simulink model "ExampleDPWM"  (R2023b)
settings: Solver=VariableStepAuto  StartTime=0.0  StopTime=0.1  FixedStep=50e-6  RelTol=1e-3
libraries: spsMosfetLib x6, spsSeriesRLCBranchLib x3, spsDCVoltageSourceLib x1, spsGroundLib x1, simulink_extras x1, spsThreePhaseVIMeasurementLib x1, spsTriangleGeneratorLib x1, spsVoltageMeasurementLib x1, sps_lib x1
settings Model: Creator=user  LastModifiedBy=user
settings DataIOCC: ReturnWorkspaceOutputs=off

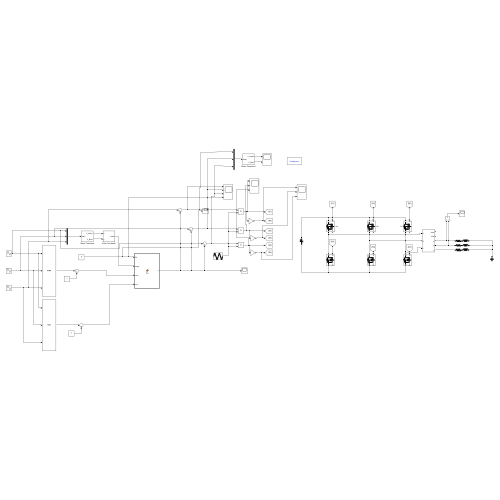
[thumbnail: Simulink's stored preview of the top-level diagram]
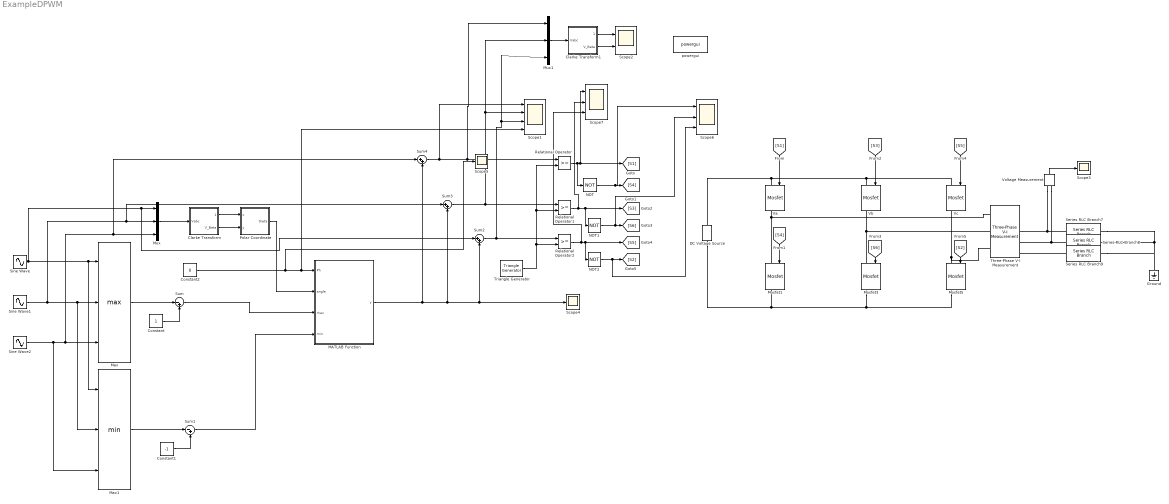
== system ExampleDPWM ==
  Clarke Transform : Subsystem
  Clarke Transform1 : Subsystem
  Constant : Constant
  Constant1 : Constant  Value=-1
  Constant2 : Constant  Value=0
  DC Voltage Source : spsDCVoltageSourceLib/DC Voltage Source  Amplitude=100  Measurements=None
  Ground : spsGroundLib/Ground  LConnTagsString=a
  MATLAB Function : MATLAB Function  TreatAsAtomicUnit=on
  Max : MinMax  Function=max  Inputs=3
  Max1 : MinMax  Inputs=3
  Mosfet1 : spsMosfetLib/Mosfet  Ron=0.1  Lon=0  Rd=0.01  Vfd=0  IC=0  Rs=1e5  Cs=inf  Measurements=on
  Mosfet3 : spsMosfetLib/Mosfet  Ron=0.1  Lon=0  Rd=0.01  Vfd=0  IC=0  Rs=1e5  Cs=inf  Measurements=on
  Mosfet5 : spsMosfetLib/Mosfet  Ron=0.1  Lon=0  Rd=0.01  Vfd=0  IC=0  Rs=1e5  Cs=inf  Measurements=on
  Mux : Mux  Inputs=3
  Mux1 : Mux  Inputs=3
  NOT : Logic  Operator=NOT  IconShape=distinctive  AllPortsSameDT=off  OutDataTypeStr=boolean
  NOT1 : Logic  Operator=NOT  IconShape=distinctive  AllPortsSameDT=off  OutDataTypeStr=boolean
  NOT2 : Logic  Operator=NOT  IconShape=distinctive  AllPortsSameDT=off  OutDataTypeStr=boolean
  Polar Coordinate : Subsystem
  Relational Operator : RelationalOperator  OutDataTypeStr=boolean  RndMeth=Simplest  InputSameDT=off
  Relational Operator1 : RelationalOperator  OutDataTypeStr=boolean  RndMeth=Simplest  InputSameDT=off
  Relational Operator2 : RelationalOperator  OutDataTypeStr=boolean  RndMeth=Simplest  InputSameDT=off
  Scope1 : Scope  NumInputPorts=4
  Scope2 : Scope  NumInputPorts=2
  Scope3 : Scope
  Scope4 : Scope
  Scope5 : Scope
  Scope6 : Scope  NumInputPorts=3
  Scope7 : Scope  NumInputPorts=3
  Series RLC Branch7 : spsSeriesRLCBranchLib/Series RLC Branch  LConnTagsString=__new0  RConnTagsString=__new0  BranchType=RL  Resistance=15  Inductance=10e-2  SetiL0=off  InitialCurrent=0  Capacitance=50e-6  Setx0=off  InitialVoltage=0  Measurements=None
  Series RLC Branch8 : spsSeriesRLCBranchLib/Series RLC Branch  LConnTagsString=__new0  RConnTagsString=__new0  BranchType=RL  Resistance=15  Inductance=10e-2  SetiL0=off  InitialCurrent=0  Capacitance=50e-6  Setx0=off  InitialVoltage=0  Measurements=None
  Series RLC Branch9 : spsSeriesRLCBranchLib/Series RLC Branch  LConnTagsString=__new0  RConnTagsString=__new0  BranchType=RL  Resistance=15  Inductance=10e-2  SetiL0=off  InitialCurrent=0  Capacitance=50e-6  Setx0=off  InitialVoltage=0  Measurements=None
  Sine Wave : Sin  Frequency=2*pi*50  SampleTime=0
  Sine Wave1 : Sin  Frequency=2*pi*50  Phase=(2*pi/3)  SampleTime=0
  Sine Wave2 : Sin  Frequency=2*pi*50  Phase=-2*pi/3  SampleTime=0
  Sum : Sum  Inputs=|-+
  Sum1 : Sum  Inputs=|-+
  Sum2 : Sum  Inputs=|++
  Sum3 : Sum  Inputs=|++
  Sum4 : Sum  Inputs=|++
  Three-Phase V-I Measurement : spsThreePhaseVIMeasurementLib/Three-Phase V-I Measurement  VoltageMeasurement=phase-to-phase  SetLabelV=off  LabelV=Vabc  Vpu=off  VpuLL=off  CurrentMeasurement=yes  SetLabelI=off  LabelI=Iabc  Ipu=off  Pbase=100e6  Vbase=500e3  OutputType=Complex  PhasorSimulation=off  PSBequivalent=0
  Triangle Generator : spsTriangleGeneratorLib/Triangle Generator  Freq=4000  Phase=90  Ts=0
  Va : spsMosfetLib/Mosfet  Ron=0.1  Lon=0  Rd=0.01  Vfd=0  IC=0  Rs=1e5  Cs=inf  Measurements=on
  Vb : spsMosfetLib/Mosfet  Ron=0.1  Lon=0  Rd=0.01  Vfd=0  IC=0  Rs=1e5  Cs=inf  Measurements=on
  Vc : spsMosfetLib/Mosfet  Ron=0.1  Lon=0  Rd=0.01  Vfd=0  IC=0  Rs=1e5  Cs=inf  Measurements=on
  Voltage Measurement : spsVoltageMeasurementLib/Voltage Measurement  PhasorSimulation=off  OutputType=Complex  PSBequivalent=0
  powergui : sps_lib/powergui  Priority=1  SimulationMode=Continuous  SampleTime=50e-6  frequency=60  Iterations=50  frequencyindice=0  Pbase=100e6  ErrMax=1e-4  UnitsV=kV  UnitsW=MW  buscounter=0  FunctionMessages=off  echomessages=off  EnableUseOfTLC=off  CurrentSourceSwitches=off  DisableSnubberDevices=off  DisableRonSwitches=off  DisableVfSwitches=off  DisplayEquations=off  AutomaticDiscreteSolvers=off  SolverType=Tustin/Backward Euler (TBE)  Interpol=off  ExternalGateDelay=off  methode=off  Ts=100  x0status=blocks  SPID=on  SwTol=0  HookPort=off  NonlinearTolerance=1e-4  nMaxIteration=100  ContinueOnMaxIteration=off  RestoreLinks=warning  ResistiveCurrentMeasurement=off  Frange=[0:2:500]  Ylog=off  Xlog=on  ShowGrid=off  save=off  variable=ZData  structure=0  ZoomFFT=off  StartTime=0.0  cycles=1  DisplayStyle=1  fundamental=60  FreqAxis=off  MaxFrequency=1000  frequencyindicesteady=1  RmsSteady=1  display=off
  wires:
  Sine Wave1/1 -> Sum3/1, Mux/2, Max1/2, Max/2
  Sine Wave2/1 -> Max1/3, Sum4/1, Mux/3, Max/3
  Max/1 -> Sum/1
  Constant/1 -> Sum/2
  Constant1/1 -> Sum1/2
  Max1/1 -> Sum1/1
  Clarke Transform/1(V_Alpha) -> Polar Coordinate/1(x)
  Clarke Transform/2(V_Beta) -> Polar Coordinate/2(y)
  Sine Wave/1 -> Sum2/1, Mux/1, Max1/1, Max/1
  Mux/1 -> Clarke Transform/1(Vabc)
  Polar Coordinate/1(theta) -> MATLAB Function/2(angle)
  Sum/1 -> MATLAB Function/3(max)
  Sum1/1 -> MATLAB Function/4(min)
  Sum3/1 -> Mux1/2, Scope1/2, Relational Operator1/1
  [S4] -> Mosfet1/1
  [S1] -> Va/1
  [S3] -> Vb/1
  [S2] -> Mosfet5/1
  [S5] -> Vc/1
  [S6] -> Mosfet3/1
  Relational Operator1/1 -> Scope7/2, [S3], NOT1/1
  Relational Operator2/1 -> Scope7/3, [S5], NOT2/1
  Triangle Generator/1 -> Relational Operator2/2, Relational Operator/2, Relational Operator1/2
  Relational Operator/1 -> Scope7/1, [S1], NOT/1
  Sum2/1 -> Mux1/3, Scope1/3, Relational Operator2/1
  NOT/1 -> Scope6/1, [S4]
  NOT1/1 -> Scope6/2, [S6]
  NOT2/1 -> Scope6/3, [S2]
  MATLAB Function/1(y) -> Sum4/2, Sum3/2, Sum2/2, Scope4/1
  Mux1/1 -> Clarke Transform1/1(Vabc)
  Clarke Transform1/1(V_Alpha) -> Scope2/1
  Clarke Transform1/2(V_Beta) -> Scope2/2
  Voltage Measurement/1 -> Scope3/1
  Constant2/1 -> Scope5/1, Scope1/4, MATLAB Function/1(Ph)
  Sum4/1 -> Scope1/1, Mux1/1, Relational Operator/1
  connections:
  Three-Phase V-I Measurement/LConn1 -- Va/RConn1 -- Mosfet1/LConn1
  Mosfet5/LConn1 -- Vc/RConn1 -- Three-Phase V-I Measurement/LConn3
  Mosfet5/RConn1 -- DC Voltage Source/LConn1 -- Mosfet1/RConn1 -- Mosfet3/RConn1
  Series RLC Branch7/RConn1 -- Series RLC Branch8/RConn1 -- Ground/LConn1 -- Series RLC Branch9/RConn1
  Vb/LConn1 -- Vc/LConn1 -- DC Voltage Source/RConn1 -- Va/LConn1
  Three-Phase V-I Measurement/LConn2 -- Vb/RConn1 -- Mosfet3/LConn1
  Series RLC Branch8/LConn1 -- Voltage Measurement/LConn2 -- Three-Phase V-I Measurement/RConn2
  Series RLC Branch7/LConn1 -- Voltage Measurement/LConn1 -- Three-Phase V-I Measurement/RConn1
  Series RLC Branch9/LConn1 -- Three-Phase V-I Measurement/RConn3

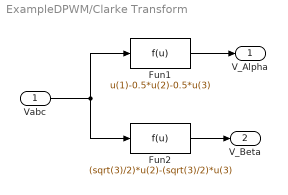
== system ExampleDPWM/Clarke Transform ==
  Vabc : Inport
  Fun1 : Fcn  Expr=u(1)-0.5*u(2)-0.5*u(3)
  Fun2 : Fcn  Expr=(sqrt(3)/2)*u(2)-(sqrt(3)/2)*u(3)
  V_Alpha : Outport
  V_Beta : Outport  Port=2
  wires:
  Fun1/1 -> V_Alpha/1
  Fun2/1 -> V_Beta/1
  Vabc/1 -> Fun1/1, Fun2/1

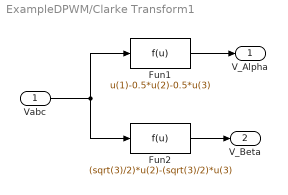
== system ExampleDPWM/Clarke Transform1 ==
  Vabc : Inport
  Fun1 : Fcn  Expr=u(1)-0.5*u(2)-0.5*u(3)
  Fun2 : Fcn  Expr=(sqrt(3)/2)*u(2)-(sqrt(3)/2)*u(3)
  V_Alpha : Outport
  V_Beta : Outport  Port=2
  wires:
  Vabc/1 -> Fun2/1, Fun1/1
  Fun2/1 -> V_Beta/1
  Fun1/1 -> V_Alpha/1

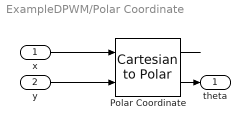
== system ExampleDPWM/Polar Coordinate ==
  x : Inport
  y : Inport  Port=2
  Polar Coordinate : simulink_extras/Transformations/Cartesian to Polar
  theta : Outport
  wires:
  y/1 -> Polar Coordinate/2
  Polar Coordinate/1 -> ?
  Polar Coordinate/2 -> theta/1
  x/1 -> Polar Coordinate/1

== matlab function ExampleDPWM/MATLAB Function ==
  data: Ph input; angle input; y output; max input; min input
function y = fcn(Ph, angle, max, min)
    angle = angle * 180 / pi;
    z = 0;
    if (angle >= (-150+Ph) && angle <= (-90+Ph)) || (angle >= (-30+Ph) && angle <= (30+Ph)) || (angle >= (90+Ph) && angle <= (150+Ph))
        z = max;
    elseif (angle >= (-90+Ph) && angle <= (-30+Ph)) || (angle >= (30+Ph) && angle <= (90+Ph)) || (angle >= (150+Ph) && angle <= (360+Ph))
        z = min;
    else 
        z = min;
    end

    y = z;
end
